simulink model "com_simulink_realim_estados_i"  (R2026a)
settings: Solver=VariableStepAuto  StopTime=Inf
libraries: instrumentseriallib x2, simulink x1
settings Model: Creator=Claudio  LastModifiedBy=Dante P

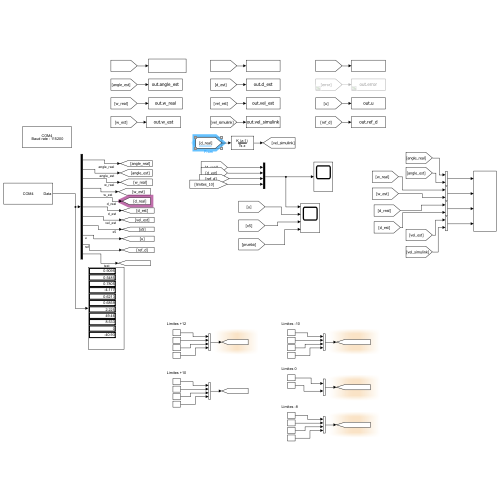
[thumbnail: Simulink's stored preview of the top-level diagram]
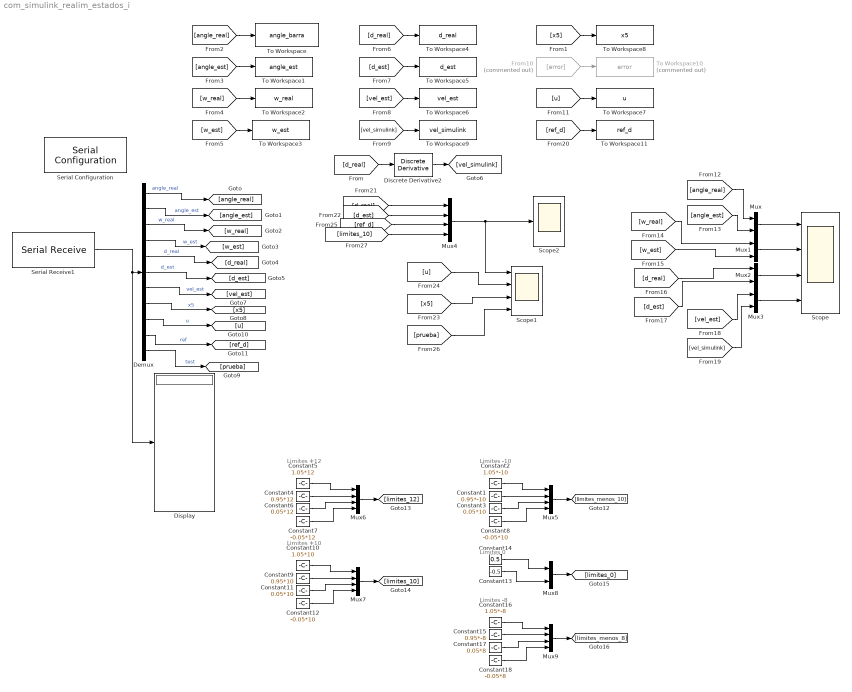
== system com_simulink_realim_estados_i ==
  note: Limites +12
  note: Limites -10
  note: Limites +10
  note: Limites 0
  note: Limites -8
  Constant1 : Constant  Value=0.95*-10  OutDataTypeStr=single  SampleTime=0.02
  Constant10 : Constant  Value=1.05*10  OutDataTypeStr=single  SampleTime=0.02
  Constant11 : Constant  Value=0.05*10  OutDataTypeStr=single  SampleTime=0.02
  Constant12 : Constant  Value=-0.05*10  OutDataTypeStr=single  SampleTime=0.02
  Constant13 : Constant  Value=-0.5  OutDataTypeStr=single  SampleTime=0.02
  Constant14 : Constant  Value=0.5  OutDataTypeStr=single  SampleTime=0.02
  Constant15 : Constant  Value=0.95*-8  OutDataTypeStr=single  SampleTime=0.02
  Constant16 : Constant  Value=1.05*-8  OutDataTypeStr=single  SampleTime=0.02
  Constant17 : Constant  Value=0.05*8  OutDataTypeStr=single  SampleTime=0.02
  Constant18 : Constant  Value=-0.05*8  OutDataTypeStr=single  SampleTime=0.02
  Constant2 : Constant  Value=1.05*-10  OutDataTypeStr=single  SampleTime=0.02
  Constant3 : Constant  Value=0.05*10  OutDataTypeStr=single  SampleTime=0.02
  Constant4 : Constant  Value=0.95*12  OutDataTypeStr=single  SampleTime=0.02
  Constant5 : Constant  Value=1.05*12  OutDataTypeStr=single  SampleTime=0.02
  Constant6 : Constant  Value=0.05*12  OutDataTypeStr=single  SampleTime=0.02
  Constant7 : Constant  Value=-0.05*12  OutDataTypeStr=single  SampleTime=0.02
  Constant8 : Constant  Value=-0.05*10  OutDataTypeStr=single  SampleTime=0.02
  Constant9 : Constant  Value=0.95*10  OutDataTypeStr=single  SampleTime=0.02
  Demux : Demux  Outputs=11
  Discrete Derivative2 : simulink/Discrete/Discrete Derivative  gainval=1.0  ICPrevScaledInput=-580  OutMin=[]  OutMax=[]  OutDataType=fixdt(1, 16)  OutScaling=2^-10  DoSatur=off
  Display : Display
  From10 : From  Commented=on  GotoTag=error
  Mux{,1..3,8} (5 alike) : Mux  Inputs=2
  Mux{4..7,9} (5 alike) : Mux
  Scope : Scope  NumInputPorts=4
      settings: TimeSpan=60  ActiveDisplayString=4  ActiveDisplayYMinimum=-23.557380199432373  ActiveDisplayYMaximum=24.947864055633545
  Scope1 : Scope  NumInputPorts=4
      settings: TimeSpan=60  ActiveDisplayYMinimum=-2.6878756284713745  ActiveDisplayYMaximum=11.965319514274597
  Scope2 : Scope
      settings: TimeSpan=60  ActiveDisplayYMinimum=-1.8749999999999998  ActiveDisplayYMaximum=11.875  DataLoggingVariableName=ScopeData2
  Serial Configuration : instrumentseriallib/Serial Configuration  Priority=-200000  PortSel=COM4  Port=COM4  ComPort=COM4  BaudRate=115200  DataBits=8  Parity=none  StopBits=1  ByteOrder=big-endian  FlowControl=none  Timeout=10  SimulateUsing=Interpreted execution  BlockInModel=on  aMode=1
  Serial Receive1 : instrumentseriallib/Serial Receive  Priority=1  PortSel=COM4  Port=COM4  ComPort=COM4  DataType=single  SaveDataType=uint8  ToggleHeader=on  Header="[ 97   98   99  100 ]"  ToggleDataSize=on  DataSize=[11 1]  ToggleTerminator=off  Terminator=<none>  CustomTerminator=[]  InputFormat=Column major  EnableBlockingMode=on  ActionDataUnavailable=Output last received value  ActionWhenDataUnavailable=Output last received value  CustomValue=0  SampleTime=0.02  SimulateUsing=Interpreted execution  BlockInModel=on  aMode=1  LibraryInUse=instrumentlib
  To Workspace : ToWorkspace  VariableName=angle_barra  SampleTime=-1
      settings: Save2DSignal=2-D array (concatenate along first dimension)
  To Workspace1 : ToWorkspace  VariableName=angle_est  SampleTime=-1
      settings: Save2DSignal=2-D array (concatenate along first dimension)
  To Workspace10 : ToWorkspace  Commented=on  VariableName=error  SampleTime=-1
      settings: Save2DSignal=2-D array (concatenate along first dimension)
  To Workspace11 : ToWorkspace  VariableName=ref_d  SampleTime=-1
      settings: Save2DSignal=2-D array (concatenate along first dimension)
  To Workspace2 : ToWorkspace  VariableName=w_real  SampleTime=-1
      settings: Save2DSignal=2-D array (concatenate along first dimension)
  To Workspace3 : ToWorkspace  VariableName=w_est  SampleTime=-1
      settings: Save2DSignal=2-D array (concatenate along first dimension)
  To Workspace4 : ToWorkspace  VariableName=d_real  SampleTime=-1
      settings: Save2DSignal=2-D array (concatenate along first dimension)
  To Workspace5 : ToWorkspace  VariableName=d_est  SampleTime=-1
      settings: Save2DSignal=2-D array (concatenate along first dimension)
  To Workspace6 : ToWorkspace  VariableName=vel_est  SampleTime=-1
      settings: Save2DSignal=2-D array (concatenate along first dimension)
  To Workspace7 : ToWorkspace  VariableName=u  SampleTime=-1
      settings: Save2DSignal=2-D array (concatenate along first dimension)
  To Workspace8 : ToWorkspace  VariableName=x5  SampleTime=-1
      settings: Save2DSignal=2-D array (concatenate along first dimension)
  To Workspace9 : ToWorkspace  VariableName=vel_simulink  SampleTime=-1
      settings: Save2DSignal=2-D array (concatenate along first dimension)
  wires:
  Demux/2 -> [angle_est]  "angle_est"
  Demux/1 -> [angle_real]  "angle_real"
  Serial Receive1/1 -> Display/1, Demux/1
  Demux/3 -> [w_real]  "w_real"
  Demux/4 -> [w_est]  "w_est"
  Mux/1 -> Scope/1
  Mux1/1 -> Scope/2
  Mux2/1 -> Scope/3
  Demux/5 -> [d_real]  "d_real"
  Demux/6 -> [d_est]  "d_est"
  Demux/7 -> [vel_est]  "vel_est"
  Mux3/1 -> Scope/4
  [d_real] -> Discrete Derivative2/1
  Discrete Derivative2/1 -> [vel_simulink]
  Demux/8 -> [x5]  "x5"
  [x5] -> To Workspace8/1
  [angle_real] -> To Workspace/1
  [angle_est] -> To Workspace1/1
  [w_real] -> To Workspace2/1
  [d_est] -> To Workspace5/1
  [w_est] -> To Workspace3/1
  [d_real] -> To Workspace4/1
  [vel_simulink] -> To Workspace9/1
  [vel_est] -> To Workspace6/1
  From10/1 -> To Workspace10/1
  [u] -> To Workspace7/1
  [angle_est] -> Mux/2
  [angle_real] -> Mux/1
  [w_est] -> Mux1/2
  [w_real] -> Mux1/1
  [d_real] -> Mux2/1
  [d_est] -> Mux2/2
  [vel_est] -> Mux3/1
  [vel_simulink] -> Mux3/2
  [d_real] -> Mux4/1
  [d_est] -> Mux4/2
  [u] -> Scope1/2
  [ref_d] -> Mux4/3
  Demux/9 -> [u]  "u"
  Demux/10 -> [ref_d]  "ref"
  [ref_d] -> To Workspace11/1
  Demux/11 -> [prueba]  "test"
  Constant5/1 -> Mux6/1
  Constant6/1 -> Mux6/3
  Constant4/1 -> Mux6/2
  Constant7/1 -> Mux6/4
  Mux6/1 -> [limites_12]
  Mux5/1 -> [limites_menos_10]
  Constant8/1 -> Mux5/4
  Constant2/1 -> Mux5/1
  Constant1/1 -> Mux5/2
  Constant3/1 -> Mux5/3
  Constant10/1 -> Mux7/1
  Constant9/1 -> Mux7/2
  Constant12/1 -> Mux7/4
  Mux7/1 -> [limites_10]
  Constant11/1 -> Mux7/3
  Constant13/1 -> Mux8/2
  Constant14/1 -> Mux8/1
  Mux8/1 -> [limites_0]
  [limites_10] -> Mux4/4
  Mux4/1 -> Scope1/1, Scope2/1
  [x5] -> Scope1/3
  [prueba] -> Scope1/4
  Constant18/1 -> Mux9/4
  Mux9/1 -> [limites_menos_8]
  Constant16/1 -> Mux9/1
  Constant17/1 -> Mux9/3
  Constant15/1 -> Mux9/2
